simulink model "SingleTrack"  (R2019b)
settings: Solver=ode1  StartTime=0  StopTime=250  FixedStep=1.0000000000000000e-003  RelTol=1e-3
InitFcn:
  | sampleTime = str2double(get_param(bdroot, 'FixedStep'));
undefined symbols (not defined in the file or in its folder): AccPedalPos, BrakePedalPos, BrakeSwitch, DiscIntNeverNeededParam, DYNA4, EngSpd, IgnitionSwitch, InitialGear, InitialSpeed, IntendedEngTrq, LeftIndicator, MainBrakePress, MaxGear, MDL, MinGear, RefAcc, RefLane, RefLatPos, RefPath, RefPathCurv, RefSpd, RefSpdPreview, RefSpdRetrospect, RightIndicator, SteeringWheelAng, SteeringWheelTrq, UserDefinedRefValue, vm_const
libraries: UtilitiesLibrary x31, simulink x18, WheelSystemModules x13, LongitudinalControllerModules x13, LateralControllerModules x7, AnimationBusselectorModules x5, EnvironmentModules x5, BasicEngineControlModules x5, MiscellaneousControlModules x5, Animation3Modules x4, AuxiliariesModules x4, ReducedTireModules x4
(part 31 of 32)

== system SingleTrack/VehicleControl/LongitudinalControl/ControlSystemsPreprocessor/Generation of Hold Data/Enabled Subsystem ==
  LongCTRL : Inport
  VehicleInfo : Inport  Port=2
  Enable : EnablePort  StatesWhenEnabling=reset  PropagateVarSize=During execution
  Add : Sum  Inputs=+-
  All zeros TD_BO_LongitudinalControlInputs : Constant  Value=0  OutDataTypeStr=Bus: TD_BO_LongitudinalControlInputs
  Bus Assignment : BusAssignment  AssignedSignals=AccPedalPos,BrakePedalPos,MainBrakePress,FrontLeftWheelBrakePress,FrontRightWheelBrakePress,RearLeftWheelBrakePress,RearRightWheelBrakePress,Rear2LeftWheelBrakePress,Rear2RightWheelBrakePress,Rear3LeftWheelBrakePress,Rear3RightWheelBrakePress,TrailerFrontLeftWheelBrakePress,TrailerFrontRightWheelBrakePress,TrailerRearLeftWheelBrakePress,TrailerRearRightWheelBrakePress,TrailerRear2LeftWheelBrakePress,TrailerRear2RightWheelBrakePress,TrailerRear3LeftWheelBrakePress,TrailerRear3RightWheelBrakePress,MinGear,MaxGear,ClutchPedalPos,ShiftingProgramSelection,IgnitionSwitch,Handbrake,ParkingLock,FrontDifferentialLock,RearDifferentialLock,Rear2DifferentialLock,Rear3DifferentialLock,TransferCaseLock,DayRunningLight,LowBeamLight,HighBeamLight,FogLampFront,FogLampRear,ESCSwitch,ABSSwitch,ACCSwitch,ACCRefSpd,AEBSwitch,RefSpd,RefSpdPreview,RefSpdRetrospect,RefAcc
  Bus Selector1 : BusSelector  OutputSignals=Chassis_VehicleBody_AbsVel[m/s],Chassis_VehicleBody_Acc_wrt_WorldSys(VehSys)[m/s**2]
  Bus Selector15 : BusSelector  OutputSignals=AccPedalPos[0_1],BrakePedalPos[0_1],MainBrakePress[Pa],FrontLeftWheelBrakePress[Pa],FrontRightWheelBrakePress[Pa],RearLeftWheelBrakePress[Pa],RearRightWheelBrakePress[Pa],Rear2LeftWheelBrakePress[Pa],Rear2RightWheelBrakePress[Pa],Rear3LeftWheelBrakePress[Pa],Rear3RightWheelBrakePress[Pa],TrailerFrontLeftWheelBrakePress[Pa],TrailerFrontRightWheelBrakePress[Pa],TrailerRearLeftWheelBrakePress[Pa],TrailerRearRightWheelBrakePress[Pa],TrailerRear2LeftWheelBrakePress[Pa],TrailerRear2RightWheelBrakePress[Pa],TrailerRear3LeftWheelBrakePress[Pa],TrailerRear3RightWheelBrakePress[Pa],MinGear[-4;20],MaxGear[-4;20],ClutchPos[0_1],ShiftingProgramSelection[-],IgnitionSwitch[0;3],Handbrake[0_1],ParkingLock[0;1],FrontDifferentialLock[0;1],RearDifferentialLock[0;1],Rear2DifferentialLock[0;1],Rear3DifferentialLock[0;1],TransferCaseLock[0;1],DayRunningLight[0;1],LowBeamLight[0;1],HighBeamLight[0;1],FogLampFront[0;1],FogLampRear[0;1],ESCSwitch[0;1],ABSSwitch[0;1],ACCSwitch[0;1],ACCRefSpd[m/s],AEBSwitch[0;1]
  Constant1 : Constant
  y component : Selector  InputPortWidth=3  IndexOptions=Index vector (dialog)  Indices=1  OutputSizes=1
  HoldData : Outport  VectorParamsAs1DForOutWhenUnconnected=off
  wires:
  Bus Selector15/21 -> Bus Assignment/22  "<MaxGear[-4;20]>"
  Bus Selector15/20 -> Bus Assignment/21  "<MinGear[-4;20]>"
  Bus Selector15/22 -> Add/2  "<ClutchPos[0_1]>"
  Bus Selector15/29 -> Bus Assignment/30  "<Rear2DifferentialLock[0;1]>"
  Bus Selector15/31 -> Bus Assignment/32  "<TransferCaseLock[0;1]>"
  Bus Selector15/6 -> Bus Assignment/7  "<RearLeftWheelBrakePress[Pa]>"
  Bus Selector15/28 -> Bus Assignment/29  "<RearDifferentialLock[0;1]>"
  Bus Selector15/17 -> Bus Assignment/18  "<TrailerRear2RightWheelBrakePress[Pa]>"
  Bus Selector15/36 -> Bus Assignment/37  "<FogLampRear[0;1]>"
  Bus Selector15/30 -> Bus Assignment/31  "<Rear3DifferentialLock[0;1]>"
  Bus Selector15/13 -> Bus Assignment/14  "<TrailerFrontRightWheelBrakePress[Pa]>"
  Bus Selector15/35 -> Bus Assignment/36  "<FogLampFront[0;1]>"
  Bus Selector15/2 -> Bus Assignment/3  "<BrakePedalPos[0_1]>"
  Bus Selector15/16 -> Bus Assignment/17  "<TrailerRear2LeftWheelBrakePress[Pa]>"
  Bus Selector15/15 -> Bus Assignment/16  "<TrailerRearRightWheelBrakePress[Pa]>"
  Bus Selector15/9 -> Bus Assignment/10  "<Rear2RightWheelBrakePress[Pa]>"
  Bus Selector15/19 -> Bus Assignment/20  "<TrailerRear3RightWheelBrakePress[Pa]>"
  Bus Selector15/23 -> Bus Assignment/24  "<ShiftingProgramSelection[-]>"
  Bus Selector15/8 -> Bus Assignment/9  "<Rear2LeftWheelBrakePress[Pa]>"
  Bus Selector15/34 -> Bus Assignment/35  "<HighBeamLight[0;1]>"
  Bus Selector15/24 -> Bus Assignment/25  "<IgnitionSwitch[0;3]>"
  Bus Selector15/33 -> Bus Assignment/34  "<LowBeamLight[0;1]>"
  Bus Selector15/26 -> Bus Assignment/27  "<ParkingLock[0;1]>"
  Bus Selector15/25 -> Bus Assignment/26  "<Handbrake[0_1]>"
  Bus Selector15/12 -> Bus Assignment/13  "<TrailerFrontLeftWheelBrakePress[Pa]>"
  Bus Selector15/10 -> Bus Assignment/11  "<Rear3LeftWheelBrakePress[Pa]>"
  Bus Selector15/14 -> Bus Assignment/15  "<TrailerRearLeftWheelBrakePress[Pa]>"
  Bus Selector15/7 -> Bus Assignment/8  "<RearRightWheelBrakePress[Pa]>"
  Bus Selector15/5 -> Bus Assignment/6  "<FrontRightWheelBrakePress[Pa]>"
  Bus Selector15/1 -> Bus Assignment/2  "<AccPedalPos[0_1]>"
  Bus Selector15/32 -> Bus Assignment/33  "<DayRunningLight[0;1]>"
  Bus Selector15/11 -> Bus Assignment/12  "<Rear3RightWheelBrakePress[Pa]>"
  Bus Selector15/3 -> Bus Assignment/4  "<MainBrakePress[Pa]>"
  Bus Selector15/27 -> Bus Assignment/28  "<FrontDifferentialLock[0;1]>"
  Bus Selector15/4 -> Bus Assignment/5  "<FrontLeftWheelBrakePress[Pa]>"
  Bus Selector15/18 -> Bus Assignment/19  "<TrailerRear3LeftWheelBrakePress[Pa]>"
  Bus Selector15/39 -> Bus Assignment/40  "<ACCSwitch[0;1]>"
  Bus Selector15/37 -> Bus Assignment/38  "<ESCSwitch[0;1]>"
  Bus Selector15/38 -> Bus Assignment/39  "<ABSSwitch[0;1]>"
  All zeros TD_BO_LongitudinalControlInputs/1 -> Bus Assignment/1
  Bus Selector15/40 -> Bus Assignment/41  "<ACCRefSpd[m/s]>"
  Bus Selector15/41 -> Bus Assignment/42  "<AEBSwitch[0;1]>"
  Bus Selector1/2 -> y component/1  "<Chassis_VehicleBody_Acc_wrt_WorldSys(VehSys)[m/s**2]>"
  Constant1/1 -> Add/1
  y component/1 -> Bus Assignment/46  "RefAcc"
  LongCTRL/1 -> Bus Selector15/1
  VehicleInfo/1 -> Bus Selector1/1
  Bus Assignment/1 -> HoldData/1
  Add/1 -> Bus Assignment/23  "ClutchPedalPos[0_1]"
  Bus Selector1/1 -> Bus Assignment/45, Bus Assignment/44, Bus Assignment/43  "<Chassis_VehicleBody_AbsVel[m/s]>"

== system SingleTrack/VehicleControl/LongitudinalControl/ControlSystemsPreprocessor/Generation of Hold Data/InitialAction Subsystem ==
  LongitudinalControlInputs : Inport
  Action Port : ActionPort  InitializeStates=reset  ActionPortLabel=case [ 1 ]:
  All zeros TD_BO_LongitudinalControlInputs : Constant  Value=0  OutDataTypeStr=Bus: TD_BO_LongitudinalControlInputs
  Bus Assignment : BusAssignment  AssignedSignals=InitialSpeed,RefSpd,RefSpdPreview,RefSpdRetrospect,InitialGear,MinGear,MaxGear
  Bus Selector1 : BusSelector  OutputSignals=InitialSpeed,InitialGear
  InitialLongitudinalControlInputs : Outport  VectorParamsAs1DForOutWhenUnconnected=off
  wires:
  Bus Selector1/2 -> Bus Assignment/6, Bus Assignment/7, Bus Assignment/8  "<InitialGear>"
  All zeros TD_BO_LongitudinalControlInputs/1 -> Bus Assignment/1
  Bus Selector1/1 -> Bus Assignment/5, Bus Assignment/4, Bus Assignment/3, Bus Assignment/2  "<InitialSpeed>"
  Bus Assignment/1 -> InitialLongitudinalControlInputs/1
  LongitudinalControlInputs/1 -> Bus Selector1/1

== system SingleTrack/VehicleControl/LongitudinalControl/ControlSystemsPreprocessor/Generation of Speed Data/Smooth Derivative ==
  note: This transfer function calculates a smooth acceleration with continuous jerk from a speed input signal.
      | The smoothing time constant T = previewTime / 2 is an input signal.
  RefSpdPrev[m/s] : Inport
  PreviewTime[s] : Inport  Port=2
  Enable : EnablePort  StatesWhenEnabling=reset
  Gain1 : Gain  Gain=0.5
  Max : MinMax  Function=max  Inputs=2
  Transfer Fcn with variable prameter : Subsystem
      mask Display: disp('num = s \n den = T^2*s^2 + 2*T*s + 1')
  limit to +/-20 : Saturate  UpperLimit=20  LowerLimit=-20
  minimum smoothing constant : Constant  Value=0.01
  SmoothedRefAcc[m/s**2] : Outport  OutputWhenDisabled=reset  InitialOutput=0  VectorParamsAs1DForOutWhenUnconnected=off
  wires:
  PreviewTime[s]/1 -> Gain1/1
  minimum smoothing constant/1 -> Max/2
  Gain1/1 -> Max/1
  RefSpdPrev[m/s]/1 -> Transfer Fcn with variable prameter/1(u)
  Max/1 -> Transfer Fcn with variable prameter/2(T)
  Transfer Fcn with variable prameter/1(y) -> limit to +/-20/1
  limit to +/-20/1 -> SmoothedRefAcc[m/s**2]/1

== system SingleTrack/VehicleControl/LongitudinalControl/ControlSystemsPreprocessor/Generation of Speed Data/Target Speed Computation Check ==
  note: TASK_LONG_ACC_BRAKE_INPUTS = 1;
      | TASK_LONG_SPEED_CONTROL = 2;
      | TASK_LONG_ACCELERATION_CONTROL = 3;
      | TASK_LONG_USER_DEFINED = 4;
  note: SOURCE_NOMINALPATH = 1;
      | 	SOURCE_LANE = 2;
      | 	SOURCE_CONSTANT = 3;
      | 	SOURCE_TABLE_DISCRETE = 4;
      | 	SOURCE_TABLE_LINEAR = 5;
      | 	SOURCE_TABLE_CUBIC = 6;
      | 	SOURCE_TABLE_HAVERSINE = 7;
      | 	SOURCE_AUTOMATIC = 8;
      | 	SOURCE_SINE_TIME = 9;
      | 	SOURCE_SINE_PATH = 10;
      | 	SOURCE_HOLD = 11;
      | 	SOURCE_EXTERNAL = 12;
      | 	SOURCE_EXTERNAL_NOMINALPATH = 13;
      | 	SOURCE_EXTERNAL_LANE = 14;
  TaskIdentifiers : Inport
  SourceIdentifiers : Inport  Port=2
  Bus Selector : BusSelector  OutputSignals=RefSpd
  Bus Selector1 : BusSelector  OutputSignals=Task
  Compare To Constant : simulink/Logic and Bit Operations/Compare To Constant  relop===  const=vm_const('TASK_LONG_SPEED_CONTROL')  OutDataTypeStr=boolean  ZeroCross=off
  Compare To Constant1 : simulink/Logic and Bit Operations/Compare To Constant  relop===  const=vm_const('SOURCE_AUTOMATIC')  OutDataTypeStr=uint8  ZeroCross=off
  Compare To Constant2 : simulink/Logic and Bit Operations/Compare To Constant  relop===  const=vm_const('TASK_LONG_USER_DEFINED')  OutDataTypeStr=boolean  ZeroCross=off
  Compare To Constant3 : simulink/Logic and Bit Operations/Compare To Constant  relop===  const=vm_const('TASK_LONG_ACCELERATION_CONTROL')  OutDataTypeStr=boolean  ZeroCross=off
  Data Type Conversion : DataTypeConversion  OutDataTypeStr=int8
  Logical Operator : Logic  AllPortsSameDT=off
  Logical Operator1 : Logic  Operator=OR  AllPortsSameDT=off
  Logical Operator3 : Logic  AllPortsSameDT=off
  Logical Operator4 : Logic  Operator=NOT  AllPortsSameDT=off
  isAutomatic : Outport  VectorParamsAs1DForOutWhenUnconnected=off
  isAccelerationControl : Outport  Port=2  VectorParamsAs1DForOutWhenUnconnected=off
  needsSmoothedDerivative : Outport  Port=3  VectorParamsAs1DForOutWhenUnconnected=off
  wires:
  Compare To Constant3/1 -> isAccelerationControl/1
  Data Type Conversion/1 -> Compare To Constant1/1
  Logical Operator1/1 -> Logical Operator/1
  Compare To Constant/1 -> Logical Operator3/1, Logical Operator1/1
  Compare To Constant2/1 -> Logical Operator1/2
  Logical Operator/1 -> isAutomatic/1
  Compare To Constant1/1 -> Logical Operator4/1, Logical Operator/2
  SourceIdentifiers/1 -> Bus Selector/1
  Bus Selector/1 -> Data Type Conversion/1  "<RefSpd>"
  Bus Selector1/1 -> Compare To Constant2/1, Compare To Constant/1, Compare To Constant3/1  "<Task>"
  TaskIdentifiers/1 -> Bus Selector1/1
  Logical Operator4/1 -> Logical Operator3/2
  Logical Operator3/1 -> needsSmoothedDerivative/1

== system SingleTrack/Vehicle/Drivetrain/DrivetrainPhysics/DrivetrainPhysicsOutputs/ClutchOutput/ClutchOutput ==
  Trq[Nm]___UNIQUE_1 : Inport  Description=|  PortDimensions=[1]
      | <name>Trq[Nm]</name>
      | <comment></comment>
  Pos[0_1]___UNIQUE_1 : Inport  Description=|  Port=2  PortDimensions=[1]
      | <name>Pos[0_1]</name>
      | <comment></comment>
  __TDD__Clutch.Pos[0_1] : Demux  Outputs=[1]
  __TDD__Clutch.Trq[Nm] : Demux  Outputs=[1]
  __TDO__Clutch : BusCreator  Inputs=2
  Clutch___UNIQUE_1 : Outport  Description=|  PortDimensions=[2]  VectorParamsAs1DForOutWhenUnconnected=off
      | <name>Trq[Nm]</name>
      | <comment></comment>
  wires:
  __TDO__Clutch/1 -> Clutch___UNIQUE_1/1  "Clutch"
  __TDD__Clutch.Pos[0_1]/1 -> __TDO__Clutch/2  "Pos[0_1]"
  Pos[0_1]___UNIQUE_1/1 -> __TDD__Clutch.Pos[0_1]/1
  __TDD__Clutch.Trq[Nm]/1 -> __TDO__Clutch/1  "Trq[Nm]"
  Trq[Nm]___UNIQUE_1/1 -> __TDD__Clutch.Trq[Nm]/1

== system SingleTrack/Vehicle/Drivetrain/DrivetrainPhysics/DrivetrainPhysicsOutputs/FrontDifferentialOutput/FrontDifferentialOutput ==
  TrqDistributionFac[0_1]___UNIQUE_1 : Inport  Description=|  PortDimensions=[1]
      | <name>TrqDistributionFac[0_1]</name>
      | <comment></comment>
  __TDD__FrontDifferential.TrqDistributionFac[0_1] : Demux  Outputs=[1]
  __TDO__FrontDifferential : BusCreator  Inputs=1
  FrontDifferential___UNIQUE_1 : Outport  Description=|  PortDimensions=[1]  VectorParamsAs1DForOutWhenUnconnected=off
      | <name>TrqDistributionFac[0_1]</name>
      | <comment></comment>
  wires:
  __TDO__FrontDifferential/1 -> FrontDifferential___UNIQUE_1/1  "FrontDifferential"
  __TDD__FrontDifferential.TrqDistributionFac[0_1]/1 -> __TDO__FrontDifferential/1  "TrqDistributionFac[0_1]"
  TrqDistributionFac[0_1]___UNIQUE_1/1 -> __TDD__FrontDifferential.TrqDistributionFac[0_1]/1

== system SingleTrack/Vehicle/Drivetrain/DrivetrainPhysics/DrivetrainPhysicsOutputs/FrontLeftShaftOutput/FrontLeftShaftOutput ==
  Trq[Nm]___UNIQUE_1 : Inport  Description=|  PortDimensions=[1]
      | <name>Trq[Nm]</name>
      | <comment></comment>
  RotSpdDifferentialOut[rad/s]___UNIQUE_1 : Inport  Description=|  Port=2  PortDimensions=[1]
      | <name>RotSpdDifferentialOut[rad/s]</name>
      | <comment></comment>
  RotAcc[rad/s**2]___UNIQUE_1 : Inport  Description=|  Port=3  PortDimensions=[1]
      | <name>RotAcc[rad/s**2]</name>
      | <comment></comment>
  DerivativeOfTrq_wrt_RotAng[Nm/rad]___UNIQUE_1 : Inport  Description=|  Port=4  PortDimensions=[1]
      | <name>DerivativeOfTrq_wrt_RotAng[Nm/rad]</name>
      | <comment></comment>
  DerivativeOfTrq_wrt_WheelSpd[Nm/(rad/s)]___UNIQUE_1 : Inport  Description=|  Port=5  PortDimensions=[1]
      | <name>DerivativeOfTrq_wrt_WheelSpd[Nm/(rad/s)]</name>
      | <comment></comment>
  AddInrt[kg*m**2]___UNIQUE_1 : Inport  Description=|  Port=6  PortDimensions=[1]
      | <name>AddInrt[kg*m**2]</name>
      | <comment></comment>
  FrictionTrq[Nm]___UNIQUE_1 : Inport  Description=|  Port=7  PortDimensions=[1]
      | <name>FrictionTrq[Nm]</name>
      | <comment></comment>
  __TDD__FrontLeftShaft.AddInrt[kg*m**2] : Demux  Outputs=[1]
  __TDD__FrontLeftShaft.DerivativeOfTrq_wrt_RotAng[Nm/rad] : Demux  Outputs=[1]
  __TDD__FrontLeftShaft.DerivativeOfTrq_wrt_WheelSpd[Nm/(rad/s)] : Demux  Outputs=[1]
  __TDD__FrontLeftShaft.FrictionTrq[Nm] : Demux  Outputs=[1]
  __TDD__FrontLeftShaft.RotAcc[rad/s**2] : Demux  Outputs=[1]
  __TDD__FrontLeftShaft.RotSpdDifferentialOut[rad/s] : Demux  Outputs=[1]
  __TDD__FrontLeftShaft.Trq[Nm] : Demux  Outputs=[1]
  __TDO__FrontLeftShaft : BusCreator  Inputs=7
  FrontLeftShaft___UNIQUE_1 : Outport  Description=|  PortDimensions=[7]  VectorParamsAs1DForOutWhenUnconnected=off
      | <name>Trq[Nm]</name>
      | <comment></comment>
  wires:
  __TDO__FrontLeftShaft/1 -> FrontLeftShaft___UNIQUE_1/1  "FrontLeftShaft"
  __TDD__FrontLeftShaft.FrictionTrq[Nm]/1 -> __TDO__FrontLeftShaft/7  "FrictionTrq[Nm]"
  FrictionTrq[Nm]___UNIQUE_1/1 -> __TDD__FrontLeftShaft.FrictionTrq[Nm]/1
  __TDD__FrontLeftShaft.AddInrt[kg*m**2]/1 -> __TDO__FrontLeftShaft/6  "AddInrt[kg*m**2]"
  AddInrt[kg*m**2]___UNIQUE_1/1 -> __TDD__FrontLeftShaft.AddInrt[kg*m**2]/1
  __TDD__FrontLeftShaft.DerivativeOfTrq_wrt_WheelSpd[Nm/(rad/s)]/1 -> __TDO__FrontLeftShaft/5  "DerivativeOfTrq_wrt_WheelSpd[Nm/(rad/s)]"
  DerivativeOfTrq_wrt_WheelSpd[Nm/(rad/s)]___UNIQUE_1/1 -> __TDD__FrontLeftShaft.DerivativeOfTrq_wrt_WheelSpd[Nm/(rad/s)]/1
  __TDD__FrontLeftShaft.DerivativeOfTrq_wrt_RotAng[Nm/rad]/1 -> __TDO__FrontLeftShaft/4  "DerivativeOfTrq_wrt_RotAng[Nm/rad]"
  DerivativeOfTrq_wrt_RotAng[Nm/rad]___UNIQUE_1/1 -> __TDD__FrontLeftShaft.DerivativeOfTrq_wrt_RotAng[Nm/rad]/1
  __TDD__FrontLeftShaft.RotAcc[rad/s**2]/1 -> __TDO__FrontLeftShaft/3  "RotAcc[rad/s**2]"
  RotAcc[rad/s**2]___UNIQUE_1/1 -> __TDD__FrontLeftShaft.RotAcc[rad/s**2]/1
  __TDD__FrontLeftShaft.RotSpdDifferentialOut[rad/s]/1 -> __TDO__FrontLeftShaft/2  "RotSpdDifferentialOut[rad/s]"
  RotSpdDifferentialOut[rad/s]___UNIQUE_1/1 -> __TDD__FrontLeftShaft.RotSpdDifferentialOut[rad/s]/1
  __TDD__FrontLeftShaft.Trq[Nm]/1 -> __TDO__FrontLeftShaft/1  "Trq[Nm]"
  Trq[Nm]___UNIQUE_1/1 -> __TDD__FrontLeftShaft.Trq[Nm]/1

== system SingleTrack/Vehicle/Drivetrain/DrivetrainPhysics/DrivetrainPhysicsOutputs/FrontRightShaftOutput/FrontRightShaftOutput ==
  Trq[Nm]___UNIQUE_1 : Inport  Description=|  PortDimensions=[1]
      | <name>Trq[Nm]</name>
      | <comment></comment>
  RotSpdDifferentialOut[rad/s]___UNIQUE_1 : Inport  Description=|  Port=2  PortDimensions=[1]
      | <name>RotSpdDifferentialOut[rad/s]</name>
      | <comment></comment>
  RotAcc[rad/s**2]___UNIQUE_1 : Inport  Description=|  Port=3  PortDimensions=[1]
      | <name>RotAcc[rad/s**2]</name>
      | <comment></comment>
  DerivativeOfTrq_wrt_RotAng[Nm/rad]___UNIQUE_1 : Inport  Description=|  Port=4  PortDimensions=[1]
      | <name>DerivativeOfTrq_wrt_RotAng[Nm/rad]</name>
      | <comment></comment>
  DerivativeOfTrq_wrt_WheelSpd[Nm/(rad/s)]___UNIQUE_1 : Inport  Description=|  Port=5  PortDimensions=[1]
      | <name>DerivativeOfTrq_wrt_WheelSpd[Nm/(rad/s)]</name>
      | <comment></comment>
  AddInrt[kg*m**2]___UNIQUE_1 : Inport  Description=|  Port=6  PortDimensions=[1]
      | <name>AddInrt[kg*m**2]</name>
      | <comment></comment>
  FrictionTrq[Nm]___UNIQUE_1 : Inport  Description=|  Port=7  PortDimensions=[1]
      | <name>FrictionTrq[Nm]</name>
      | <comment></comment>
  __TDD__FrontRightShaft.AddInrt[kg*m**2] : Demux  Outputs=[1]
  __TDD__FrontRightShaft.DerivativeOfTrq_wrt_RotAng[Nm/rad] : Demux  Outputs=[1]
  __TDD__FrontRightShaft.DerivativeOfTrq_wrt_WheelSpd[Nm/(rad/s)] : Demux  Outputs=[1]
  __TDD__FrontRightShaft.FrictionTrq[Nm] : Demux  Outputs=[1]
  __TDD__FrontRightShaft.RotAcc[rad/s**2] : Demux  Outputs=[1]
  __TDD__FrontRightShaft.RotSpdDifferentialOut[rad/s] : Demux  Outputs=[1]
  __TDD__FrontRightShaft.Trq[Nm] : Demux  Outputs=[1]
  __TDO__FrontRightShaft : BusCreator  Inputs=7
  FrontRightShaft___UNIQUE_1 : Outport  Description=|  PortDimensions=[7]  VectorParamsAs1DForOutWhenUnconnected=off
      | <name>Trq[Nm]</name>
      | <comment></comment>
  wires:
  __TDO__FrontRightShaft/1 -> FrontRightShaft___UNIQUE_1/1  "FrontRightShaft"
  __TDD__FrontRightShaft.FrictionTrq[Nm]/1 -> __TDO__FrontRightShaft/7  "FrictionTrq[Nm]"
  FrictionTrq[Nm]___UNIQUE_1/1 -> __TDD__FrontRightShaft.FrictionTrq[Nm]/1
  __TDD__FrontRightShaft.AddInrt[kg*m**2]/1 -> __TDO__FrontRightShaft/6  "AddInrt[kg*m**2]"
  AddInrt[kg*m**2]___UNIQUE_1/1 -> __TDD__FrontRightShaft.AddInrt[kg*m**2]/1
  __TDD__FrontRightShaft.DerivativeOfTrq_wrt_WheelSpd[Nm/(rad/s)]/1 -> __TDO__FrontRightShaft/5  "DerivativeOfTrq_wrt_WheelSpd[Nm/(rad/s)]"
  DerivativeOfTrq_wrt_WheelSpd[Nm/(rad/s)]___UNIQUE_1/1 -> __TDD__FrontRightShaft.DerivativeOfTrq_wrt_WheelSpd[Nm/(rad/s)]/1
  __TDD__FrontRightShaft.DerivativeOfTrq_wrt_RotAng[Nm/rad]/1 -> __TDO__FrontRightShaft/4  "DerivativeOfTrq_wrt_RotAng[Nm/rad]"
  DerivativeOfTrq_wrt_RotAng[Nm/rad]___UNIQUE_1/1 -> __TDD__FrontRightShaft.DerivativeOfTrq_wrt_RotAng[Nm/rad]/1
  __TDD__FrontRightShaft.RotAcc[rad/s**2]/1 -> __TDO__FrontRightShaft/3  "RotAcc[rad/s**2]"
  RotAcc[rad/s**2]___UNIQUE_1/1 -> __TDD__FrontRightShaft.RotAcc[rad/s**2]/1
  __TDD__FrontRightShaft.RotSpdDifferentialOut[rad/s]/1 -> __TDO__FrontRightShaft/2  "RotSpdDifferentialOut[rad/s]"
  RotSpdDifferentialOut[rad/s]___UNIQUE_1/1 -> __TDD__FrontRightShaft.RotSpdDifferentialOut[rad/s]/1
  __TDD__FrontRightShaft.Trq[Nm]/1 -> __TDO__FrontRightShaft/1  "Trq[Nm]"
  Trq[Nm]___UNIQUE_1/1 -> __TDD__FrontRightShaft.Trq[Nm]/1

== system SingleTrack/Vehicle/Drivetrain/DrivetrainPhysics/DrivetrainPhysicsOutputs/RearDifferentialOutput/RearDifferentialOutput ==
  TrqDistributionFac[0_1]___UNIQUE_1 : Inport  Description=|  PortDimensions=[1]
      | <name>TrqDistributionFac[0_1]</name>
      | <comment></comment>
  __TDD__RearDifferential.TrqDistributionFac[0_1] : Demux  Outputs=[1]
  __TDO__RearDifferential : BusCreator  Inputs=1
  RearDifferential___UNIQUE_1 : Outport  Description=|  PortDimensions=[1]  VectorParamsAs1DForOutWhenUnconnected=off
      | <name>TrqDistributionFac[0_1]</name>
      | <comment></comment>
  wires:
  __TDO__RearDifferential/1 -> RearDifferential___UNIQUE_1/1  "RearDifferential"
  __TDD__RearDifferential.TrqDistributionFac[0_1]/1 -> __TDO__RearDifferential/1  "TrqDistributionFac[0_1]"
  TrqDistributionFac[0_1]___UNIQUE_1/1 -> __TDD__RearDifferential.TrqDistributionFac[0_1]/1

== system SingleTrack/Vehicle/Drivetrain/DrivetrainPhysics/DrivetrainPhysicsOutputs/RearLeftShaftOutput/RearLeftShaftOutput ==
  Trq[Nm]___UNIQUE_1 : Inport  Description=|  PortDimensions=[1]
      | <name>Trq[Nm]</name>
      | <comment></comment>
  RotSpdDifferentialOut[rad/s]___UNIQUE_1 : Inport  Description=|  Port=2  PortDimensions=[1]
      | <name>RotSpdDifferentialOut[rad/s]</name>
      | <comment></comment>
  RotAcc[rad/s**2]___UNIQUE_1 : Inport  Description=|  Port=3  PortDimensions=[1]
      | <name>RotAcc[rad/s**2]</name>
      | <comment></comment>
  DerivativeOfTrq_wrt_RotAng[Nm/rad]___UNIQUE_1 : Inport  Description=|  Port=4  PortDimensions=[1]
      | <name>DerivativeOfTrq_wrt_RotAng[Nm/rad]</name>
      | <comment></comment>
  DerivativeOfTrq_wrt_WheelSpd[Nm/(rad/s)]___UNIQUE_1 : Inport  Description=|  Port=5  PortDimensions=[1]
      | <name>DerivativeOfTrq_wrt_WheelSpd[Nm/(rad/s)]</name>
      | <comment></comment>
  AddInrt[kg*m**2]___UNIQUE_1 : Inport  Description=|  Port=6  PortDimensions=[1]
      | <name>AddInrt[kg*m**2]</name>
      | <comment></comment>
  FrictionTrq[Nm]___UNIQUE_1 : Inport  Description=|  Port=7  PortDimensions=[1]
      | <name>FrictionTrq[Nm]</name>
      | <comment></comment>
  __TDD__RearLeftShaft.AddInrt[kg*m**2] : Demux  Outputs=[1]
  __TDD__RearLeftShaft.DerivativeOfTrq_wrt_RotAng[Nm/rad] : Demux  Outputs=[1]
  __TDD__RearLeftShaft.DerivativeOfTrq_wrt_WheelSpd[Nm/(rad/s)] : Demux  Outputs=[1]
  __TDD__RearLeftShaft.FrictionTrq[Nm] : Demux  Outputs=[1]
  __TDD__RearLeftShaft.RotAcc[rad/s**2] : Demux  Outputs=[1]
  __TDD__RearLeftShaft.RotSpdDifferentialOut[rad/s] : Demux  Outputs=[1]
  __TDD__RearLeftShaft.Trq[Nm] : Demux  Outputs=[1]
  __TDO__RearLeftShaft : BusCreator  Inputs=7
  RearLeftShaft___UNIQUE_1 : Outport  Description=|  PortDimensions=[7]  VectorParamsAs1DForOutWhenUnconnected=off
      | <name>Trq[Nm]</name>
      | <comment></comment>
  wires:
  __TDO__RearLeftShaft/1 -> RearLeftShaft___UNIQUE_1/1  "RearLeftShaft"
  __TDD__RearLeftShaft.FrictionTrq[Nm]/1 -> __TDO__RearLeftShaft/7  "FrictionTrq[Nm]"
  FrictionTrq[Nm]___UNIQUE_1/1 -> __TDD__RearLeftShaft.FrictionTrq[Nm]/1
  __TDD__RearLeftShaft.AddInrt[kg*m**2]/1 -> __TDO__RearLeftShaft/6  "AddInrt[kg*m**2]"
  AddInrt[kg*m**2]___UNIQUE_1/1 -> __TDD__RearLeftShaft.AddInrt[kg*m**2]/1
  __TDD__RearLeftShaft.DerivativeOfTrq_wrt_WheelSpd[Nm/(rad/s)]/1 -> __TDO__RearLeftShaft/5  "DerivativeOfTrq_wrt_WheelSpd[Nm/(rad/s)]"
  DerivativeOfTrq_wrt_WheelSpd[Nm/(rad/s)]___UNIQUE_1/1 -> __TDD__RearLeftShaft.DerivativeOfTrq_wrt_WheelSpd[Nm/(rad/s)]/1
  __TDD__RearLeftShaft.DerivativeOfTrq_wrt_RotAng[Nm/rad]/1 -> __TDO__RearLeftShaft/4  "DerivativeOfTrq_wrt_RotAng[Nm/rad]"
  DerivativeOfTrq_wrt_RotAng[Nm/rad]___UNIQUE_1/1 -> __TDD__RearLeftShaft.DerivativeOfTrq_wrt_RotAng[Nm/rad]/1
  __TDD__RearLeftShaft.RotAcc[rad/s**2]/1 -> __TDO__RearLeftShaft/3  "RotAcc[rad/s**2]"
  RotAcc[rad/s**2]___UNIQUE_1/1 -> __TDD__RearLeftShaft.RotAcc[rad/s**2]/1
  __TDD__RearLeftShaft.RotSpdDifferentialOut[rad/s]/1 -> __TDO__RearLeftShaft/2  "RotSpdDifferentialOut[rad/s]"
  RotSpdDifferentialOut[rad/s]___UNIQUE_1/1 -> __TDD__RearLeftShaft.RotSpdDifferentialOut[rad/s]/1
  __TDD__RearLeftShaft.Trq[Nm]/1 -> __TDO__RearLeftShaft/1  "Trq[Nm]"
  Trq[Nm]___UNIQUE_1/1 -> __TDD__RearLeftShaft.Trq[Nm]/1

== system SingleTrack/Vehicle/Drivetrain/DrivetrainPhysics/DrivetrainPhysicsOutputs/RearRightShaftOutput/RearRightShaftOutput ==
  Trq[Nm]___UNIQUE_1 : Inport  Description=|  PortDimensions=[1]
      | <name>Trq[Nm]</name>
      | <comment></comment>
  RotSpdDifferentialOut[rad/s]___UNIQUE_1 : Inport  Description=|  Port=2  PortDimensions=[1]
      | <name>RotSpdDifferentialOut[rad/s]</name>
      | <comment></comment>
  RotAcc[rad/s**2]___UNIQUE_1 : Inport  Description=|  Port=3  PortDimensions=[1]
      | <name>RotAcc[rad/s**2]</name>
      | <comment></comment>
  DerivativeOfTrq_wrt_RotAng[Nm/rad]___UNIQUE_1 : Inport  Description=|  Port=4  PortDimensions=[1]
      | <name>DerivativeOfTrq_wrt_RotAng[Nm/rad]</name>
      | <comment></comment>
  DerivativeOfTrq_wrt_WheelSpd[Nm/(rad/s)]___UNIQUE_1 : Inport  Description=|  Port=5  PortDimensions=[1]
      | <name>DerivativeOfTrq_wrt_WheelSpd[Nm/(rad/s)]</name>
      | <comment></comment>
  AddInrt[kg*m**2]___UNIQUE_1 : Inport  Description=|  Port=6  PortDimensions=[1]
      | <name>AddInrt[kg*m**2]</name>
      | <comment></comment>
  FrictionTrq[Nm]___UNIQUE_1 : Inport  Description=|  Port=7  PortDimensions=[1]
      | <name>FrictionTrq[Nm]</name>
      | <comment></comment>
  __TDD__RearRightShaft.AddInrt[kg*m**2] : Demux  Outputs=[1]
  __TDD__RearRightShaft.DerivativeOfTrq_wrt_RotAng[Nm/rad] : Demux  Outputs=[1]
  __TDD__RearRightShaft.DerivativeOfTrq_wrt_WheelSpd[Nm/(rad/s)] : Demux  Outputs=[1]
  __TDD__RearRightShaft.FrictionTrq[Nm] : Demux  Outputs=[1]
  __TDD__RearRightShaft.RotAcc[rad/s**2] : Demux  Outputs=[1]
  __TDD__RearRightShaft.RotSpdDifferentialOut[rad/s] : Demux  Outputs=[1]
  __TDD__RearRightShaft.Trq[Nm] : Demux  Outputs=[1]
  __TDO__RearRightShaft : BusCreator  Inputs=7
  RearRightShaft___UNIQUE_1 : Outport  Description=|  PortDimensions=[7]  VectorParamsAs1DForOutWhenUnconnected=off
      | <name>Trq[Nm]</name>
      | <comment></comment>
  wires:
  __TDO__RearRightShaft/1 -> RearRightShaft___UNIQUE_1/1  "RearRightShaft"
  __TDD__RearRightShaft.FrictionTrq[Nm]/1 -> __TDO__RearRightShaft/7  "FrictionTrq[Nm]"
  FrictionTrq[Nm]___UNIQUE_1/1 -> __TDD__RearRightShaft.FrictionTrq[Nm]/1
  __TDD__RearRightShaft.AddInrt[kg*m**2]/1 -> __TDO__RearRightShaft/6  "AddInrt[kg*m**2]"
  AddInrt[kg*m**2]___UNIQUE_1/1 -> __TDD__RearRightShaft.AddInrt[kg*m**2]/1
  __TDD__RearRightShaft.DerivativeOfTrq_wrt_WheelSpd[Nm/(rad/s)]/1 -> __TDO__RearRightShaft/5  "DerivativeOfTrq_wrt_WheelSpd[Nm/(rad/s)]"
  DerivativeOfTrq_wrt_WheelSpd[Nm/(rad/s)]___UNIQUE_1/1 -> __TDD__RearRightShaft.DerivativeOfTrq_wrt_WheelSpd[Nm/(rad/s)]/1
  __TDD__RearRightShaft.DerivativeOfTrq_wrt_RotAng[Nm/rad]/1 -> __TDO__RearRightShaft/4  "DerivativeOfTrq_wrt_RotAng[Nm/rad]"
  DerivativeOfTrq_wrt_RotAng[Nm/rad]___UNIQUE_1/1 -> __TDD__RearRightShaft.DerivativeOfTrq_wrt_RotAng[Nm/rad]/1
  __TDD__RearRightShaft.RotAcc[rad/s**2]/1 -> __TDO__RearRightShaft/3  "RotAcc[rad/s**2]"
  RotAcc[rad/s**2]___UNIQUE_1/1 -> __TDD__RearRightShaft.RotAcc[rad/s**2]/1
  __TDD__RearRightShaft.RotSpdDifferentialOut[rad/s]/1 -> __TDO__RearRightShaft/2  "RotSpdDifferentialOut[rad/s]"
  RotSpdDifferentialOut[rad/s]___UNIQUE_1/1 -> __TDD__RearRightShaft.RotSpdDifferentialOut[rad/s]/1
  __TDD__RearRightShaft.Trq[Nm]/1 -> __TDO__RearRightShaft/1  "Trq[Nm]"
  Trq[Nm]___UNIQUE_1/1 -> __TDD__RearRightShaft.Trq[Nm]/1

== system SingleTrack/Vehicle/Drivetrain/DrivetrainPhysics/DrivetrainPhysicsOutputs/TransferCaseOutput/TransferCaseOutput ==
  TrqDistributionFac[0_1]___UNIQUE_1 : Inport  Description=|  PortDimensions=[1]
      | <name>TrqDistributionFac[0_1]</name>
      | <comment></comment>
  __TDD__TransferCase.TrqDistributionFac[0_1] : Demux  Outputs=[1]
  __TDO__TransferCase : BusCreator  Inputs=1
  TransferCase___UNIQUE_1 : Outport  Description=|  PortDimensions=[1]  VectorParamsAs1DForOutWhenUnconnected=off
      | <name>TrqDistributionFac[0_1]</name>
      | <comment></comment>
  wires:
  __TDO__TransferCase/1 -> TransferCase___UNIQUE_1/1  "TransferCase"
  __TDD__TransferCase.TrqDistributionFac[0_1]/1 -> __TDO__TransferCase/1  "TrqDistributionFac[0_1]"
  TrqDistributionFac[0_1]___UNIQUE_1/1 -> __TDD__TransferCase.TrqDistributionFac[0_1]/1

== system SingleTrack/Vehicle/Drivetrain/DrivetrainPhysics/DrivetrainPhysicsOutputs/TransmissionOutput/TransmissionOutput ==
  NumFwdGears[-]___UNIQUE_1 : Inport  Description=|  PortDimensions=[1]
      | <name>NumFwdGears[-]</name>
      | <comment></comment>
  Type[-]___UNIQUE_1 : Inport  Description=|  Port=2  PortDimensions=[1]
      | <name>Type[-]</name>
      | <comment></comment>
  Gear[-4;20]___UNIQUE_1 : Inport  Description=|  Port=3  PortDimensions=[1]
      | <name>Gear[-4;20]</name>
      | <comment></comment>
  InSpd[rad/s]___UNIQUE_1 : Inport  Description=|  Port=4  PortDimensions=[1]
      | <name>InSpd[rad/s]</name>
      | <comment></comment>
  OutSpd[rad/s]___UNIQUE_1 : Inport  Description=|  Port=5  PortDimensions=[1]
      | <name>OutSpd[rad/s]</name>
      | <comment></comment>
  GearChangeTimeConst[s]___UNIQUE_1 : Inport  Description=|  Port=6  PortDimensions=[1]
      | <name>GearChangeTimeConst[s]</name>
      | <comment></comment>
  __TDD__Transmission.GearChangeTimeConst[s] : Demux  Outputs=[1]
  __TDD__Transmission.Gear[-4;20] : Demux  Outputs=[1]
  __TDD__Transmission.InSpd[rad/s] : Demux  Outputs=[1]
  __TDD__Transmission.NumFwdGears[-] : Demux  Outputs=[1]
  __TDD__Transmission.OutSpd[rad/s] : Demux  Outputs=[1]
  __TDD__Transmission.Type[-] : Demux  Outputs=[1]
  __TDO__Transmission : BusCreator  Inputs=6
  Transmission___UNIQUE_1 : Outport  Description=|  PortDimensions=[6]  VectorParamsAs1DForOutWhenUnconnected=off
      | <name>NumFwdGears[-]</name>
      | <comment></comment>
  wires:
  __TDO__Transmission/1 -> Transmission___UNIQUE_1/1  "Transmission"
  __TDD__Transmission.GearChangeTimeConst[s]/1 -> __TDO__Transmission/6  "GearChangeTimeConst[s]"
  GearChangeTimeConst[s]___UNIQUE_1/1 -> __TDD__Transmission.GearChangeTimeConst[s]/1
  __TDD__Transmission.OutSpd[rad/s]/1 -> __TDO__Transmission/5  "OutSpd[rad/s]"
  OutSpd[rad/s]___UNIQUE_1/1 -> __TDD__Transmission.OutSpd[rad/s]/1
  __TDD__Transmission.InSpd[rad/s]/1 -> __TDO__Transmission/4  "InSpd[rad/s]"
  InSpd[rad/s]___UNIQUE_1/1 -> __TDD__Transmission.InSpd[rad/s]/1
  __TDD__Transmission.Gear[-4;20]/1 -> __TDO__Transmission/3  "Gear[-4;20]"
  Gear[-4;20]___UNIQUE_1/1 -> __TDD__Transmission.Gear[-4;20]/1
  __TDD__Transmission.Type[-]/1 -> __TDO__Transmission/2  "Type[-]"
  Type[-]___UNIQUE_1/1 -> __TDD__Transmission.Type[-]/1
  __TDD__Transmission.NumFwdGears[-]/1 -> __TDO__Transmission/1  "NumFwdGears[-]"
  NumFwdGears[-]___UNIQUE_1/1 -> __TDD__Transmission.NumFwdGears[-]/1

== system SingleTrack/VehicleControl/LateralControl/Disabled LateralControl/ControlSystems/Control Systems Parameters/CurvatureControl ==
  DynaModuleInfo : Subsystem  Tag=DynaModuleInfo
      mask init:
      | data = get_param(gcb, 'UserData');
      mask Display: disp(['Type = ', data.type, '\nName = ', char(data.name)]);

== system SingleTrack/VehicleControl/LateralControl/Disabled LateralControl/ControlSystems/Control Systems Parameters/PathControl ==
  DynaModuleInfo : Subsystem  Tag=DynaModuleInfo
      mask init:
      | data = get_param(gcb, 'UserData');
      mask Display: disp(['Type = ', data.type, '\nName = ', char(data.name)]);

== system SingleTrack/VehicleControl/LateralControl/Disabled LateralControl/ControlSystems/Lateral Controller/User-Defined Control ==
  UserDefinedControl : Subsystem
      settings: CopyFcn=DYNA4.Internal.ModelCallbacks.Modules.UpdateMaskParameters(gcb);  DeleteFcn=dm_close_block_mask  ModelCloseFcn=dm_close_block_mask  NameChangeFcn=DYNA4.Internal.ModelCallbacks.Modules.UpdateMaskParameters(gcb);  OpenFcn=dm_open_block_mask('vm_dflt_vehiclecontrol_user_defined_lateral_control');

== system SingleTrack/VehicleControl/LateralControl/Disabled LateralControl/ControlSystemsPreprocessor/Maneuver/DynaModuleInfo ==

== system SingleTrack/VehicleControl/LateralControl/Enabled LateralControl/ControlSystems/Lateral Controller/Initialization ==
  Action Port : ActionPort  InitializeStates=reset  PropagateVarSize=During execution  ActionPortLabel=default:
  Bus Creator : BusCreator  Inputs=3
  Constant : Constant  Value=0
  Constant1 : Constant  Value=0
  Constant2 : Constant  Value=0
  SteeringWheelDemands : Outport  VectorParamsAs1DForOutWhenUnconnected=off
  wires:
  Constant2/1 -> Bus Creator/3  "SteeringWheelInputSwitch[-]"
  Constant1/1 -> Bus Creator/2  "SteeringWheelTrq[Nm]"
  Bus Creator/1 -> SteeringWheelDemands/1
  Constant/1 -> Bus Creator/1  "SteeringWheelAng[rad]"

== system SingleTrack/VehicleControl/LateralControl/Enabled LateralControl/ControlSystems/Lateral Controller/Path and Curvature Control ==
  ControlInputs : Inport
  ControllerParameters : Inport  Port=2
  VehicleInfo : Inport  Port=3
  Action Port : ActionPort  InitializeStates=reset  PropagateVarSize=During execution  ActionPortLabel=case [ 3 4 ]:
  Bus Creator : BusCreator  Inputs=3
  Bus Selector1 : BusSelector  OutputSignals=Chassis_FrontAxle_Steering_SteeringWheelTrq[Nm]
  Constant1 : Constant  Value=0
  Gain : Gain
  PathControl : LateralControllerModules/PathControl  Tag=vedynaPathCtrlMask  local_comp_inst=1  system_comp_inst=1  sample_time=-1
  required by merge block : SignalConversion  OverrideOpt=off
  SteeringWheelDemands : Outport  VectorParamsAs1DForOutWhenUnconnected=off
  wires:
  Gain/1 -> Bus Creator/2  "SteeringWheelTrq[Nm]"
  Bus Selector1/1 -> Gain/1  "<Chassis_FrontAxle_Steering_SteeringWheelTrq[Nm]>"
  required by merge block/1 -> Bus Creator/1  "SteeringWheelAng[rad]"
  Constant1/1 -> Bus Creator/3  "SteeringWheelInputSwitch[-]"
  Bus Creator/1 -> SteeringWheelDemands/1
  PathControl/1 -> required by merge block/1
  ControllerParameters/1 -> PathControl/2
  ControlInputs/1 -> PathControl/1
  VehicleInfo/1 -> PathControl/3, Bus Selector1/1

== system SingleTrack/VehicleControl/LateralControl/Enabled LateralControl/ControlSystems/Lateral Controller/Steering Wheel Angle Input ==
  ControlInputs : Inport
  VehicleInfo : Inport  Port=2
  Action Port : ActionPort  InitializeStates=reset  PropagateVarSize=During execution  ActionPortLabel=case [ 1 ]:
  Bus Creator : BusCreator  Inputs=3
  Bus Selector : BusSelector  OutputSignals=SteeringWheelAng
  Bus Selector1 : BusSelector  OutputSignals=Chassis_FrontAxle_Steering_SteeringWheelTrq[Nm]
  Constant1 : Constant  Value=0
  Gain : Gain
  required by merge block : SignalConversion  OverrideOpt=off
  SteeringWheelDemands : Outport  VectorParamsAs1DForOutWhenUnconnected=off
  wires:
  Gain/1 -> Bus Creator/2  "SteeringWheelTrq[Nm]"
  VehicleInfo/1 -> Bus Selector1/1
  Constant1/1 -> Bus Creator/3  "SteeringWheelInputSwitch[-]"
  Bus Selector1/1 -> Gain/1  "<Chassis_FrontAxle_Steering_SteeringWheelTrq[Nm]>"
  Bus Creator/1 -> SteeringWheelDemands/1
  required by merge block/1 -> Bus Creator/1  "SteeringWheelAng[rad]"
  Bus Selector/1 -> required by merge block/1  "<SteeringWheelAng>"
  ControlInputs/1 -> Bus Selector/1

== system SingleTrack/VehicleControl/LateralControl/Enabled LateralControl/ControlSystems/Lateral Controller/Steering Wheel Torque Input ==
  ControlInputs : Inport
  VehicleInfo : Inport  Port=2
  Action Port : ActionPort  InitializeStates=reset  PropagateVarSize=During execution  ActionPortLabel=case [ 2 ]:
  Bus Creator : BusCreator  Inputs=3
  Bus Selector : BusSelector  OutputSignals=SteeringWheelTrq
  Bus Selector1 : BusSelector  OutputSignals=Chassis_FrontAxle_Steering_SteeringWheelAng[rad]
  Constant1 : Constant
  Gain : Gain
  required by merge block : SignalConversion  OverrideOpt=off
  SteeringWheelDemands : Outport  VectorParamsAs1DForOutWhenUnconnected=off
  wires:
  Gain/1 -> Bus Creator/1  "SteeringWheelAng[rad]"
  required by merge block/1 -> Bus Creator/2  "SteeringWheelTrq[Nm]"
  VehicleInfo/1 -> Bus Selector1/1
  Bus Selector/1 -> required by merge block/1  "<SteeringWheelTrq>"
  ControlInputs/1 -> Bus Selector/1
  Bus Selector1/1 -> Gain/1  "<Chassis_FrontAxle_Steering_SteeringWheelAng[rad]>"
  Bus Creator/1 -> SteeringWheelDemands/1
  Constant1/1 -> Bus Creator/3  "SteeringWheelInputSwitch[-]"

== system SingleTrack/VehicleControl/LateralControl/Enabled LateralControl/ControlSystems/Lateral Controller/User-Defined Control ==
  ControlInputs : Inport
  VehicleInfo : Inport  Port=2
  SourceIdentifiers : Inport  Port=3
  SubtaskIdentifiers : Inport  Port=4
  Action Port : ActionPort  InitializeStates=reset  PropagateVarSize=During execution  ActionPortLabel=case [ 5 ]:
  Bus Creator : BusCreator  Inputs=3
  Bus Selector1 : BusSelector  OutputSignals=UserDefinedRefValue
  Bus Selector2 : BusSelector  OutputSignals=Chassis_FrontAxle_Steering_SteeringWheelTrq[Nm]
  Constant1 : Constant  Value=0
  Gain : Gain
  UserDefinedControl : LateralControllerModules/UserDefinedLateralControl  DATA_NODE=MDL.VehicleControl.LateralControl.ControlSystems.UserDefinedControl  SteeringWheelAngle=MDL.VehicleControl.LateralControl.ControlSystems.UserDefinedControl.SteeringWheelAng
  SteeringWheelDemands : Outport  VectorParamsAs1DForOutWhenUnconnected=off
  UserDefinedRefValue[-] : Outport  Port=2  PortDimensions=1  OutputWhenDisabled=reset  InitialOutput=0  VectorParamsAs1DForOutWhenUnconnected=off
  wires:
  Gain/1 -> Bus Creator/2  "SteeringWheelTrq[Nm]"
  Bus Selector2/1 -> Gain/1  "<Chassis_FrontAxle_Steering_SteeringWheelTrq[Nm]>"
  Constant1/1 -> Bus Creator/3  "SteeringWheelInputSwitch[-]"
  Bus Creator/1 -> SteeringWheelDemands/1
  UserDefinedControl/1 -> Bus Creator/1  "SteeringWheelAng[rad]"
  Bus Selector1/1 -> UserDefinedRefValue[-]/1  "<UserDefinedRefValue>"
  SubtaskIdentifiers/1 -> UserDefinedControl/1
  VehicleInfo/1 -> UserDefinedControl/4, Bus Selector2/1
  SourceIdentifiers/1 -> UserDefinedControl/2
  ControlInputs/1 -> Bus Selector1/1, UserDefinedControl/3

== system SingleTrack/VehicleControl/LateralControl/Enabled LateralControl/ControlSystemsPreprocessor/External Presetting of Controller /Presetting Source Identifiers ==
  note: SOURCE_NOMINALPATH = 1;
      | 	SOURCE_LANE = 2;
      | 	SOURCE_CONSTANT = 3;
      | 	SOURCE_TABLE_DISCRETE = 4;
      | 	SOURCE_TABLE_LINEAR = 5;
      | 	SOURCE_TABLE_CUBIC = 6;
      | 	SOURCE_TABLE_HAVERSINE = 7;
      | 	SOURCE_AUTOMATIC = 8;
      | 	SOURCE_SINE_TIME = 9;
      | 	SOURCE_SINE_PATH = 10;
      | 	SOURCE_HOLD = 11;
      | 	SOURCE_EXTERNAL = 12;
      | 	SOURCE_EXTERNAL_NOMINALPATH = 13;
      | 	SOURCE_EXTERNAL_LANE = 14;
  "ExternalControlVariablesEnforced " : Inport
  SourceIdentifiers : Inport  Port=2
  Bus Selector : BusSelector  OutputSignals=CTRL_LateralControl_RefPathEnforced,CTRL_LateralControl_RefLaneEnforced,CTRL_LateralControl_RefLatPosEnforced,CTRL_LateralControl_RefCurvEnforced,CTRL_LateralControl_UserDefinedRefValueEnforced
  Bus Selector6 : BusSelector  OutputSignals=RefPath,RefLane,RefLatPos,RefPathCurv,UserDefinedRefValue
  PathCtrl_Path : BusAssignment  AssignedSignals=RefPath,RefLane,RefLatPos,RefPathCurv,UserDefinedRefValue
  RefLaneExternal : Constant  Value=vm_const('SOURCE_EXTERNAL_LANE')
  RefLatPosExternal : Constant  Value=vm_const('SOURCE_EXTERNAL')
  RefPathCurvExternal : Constant  Value=vm_const('SOURCE_EXTERNAL')
  RefPathExternal : Constant  Value=vm_const('SOURCE_EXTERNAL_NOMINALPATH')
  Switch{1..2,5..7} (5 alike) : Switch  Criteria=u2 > Threshold
  UserDefinedRefValueExternal : Constant  Value=vm_const('SOURCE_EXTERNAL')
  ModifiedSourceIdentifiers : Outport  VectorParamsAs1DForOutWhenUnconnected=off
  wires:
  Bus Selector6/5 -> Switch2/3  "<UserDefinedRefValue>"
  Bus Selector6/4 -> Switch1/3  "<RefPathCurv>"
  Bus Selector6/3 -> Switch7/3  "<RefLatPos>"
  Bus Selector6/2 -> Switch6/3  "<RefLane>"
  Bus Selector6/1 -> Switch5/3  "<RefPath>"
  Switch2/1 -> PathCtrl_Path/6
  Switch1/1 -> PathCtrl_Path/5
  Switch7/1 -> PathCtrl_Path/4
  Switch6/1 -> PathCtrl_Path/3
  Switch5/1 -> PathCtrl_Path/2
  PathCtrl_Path/1 -> ModifiedSourceIdentifiers/1
  Bus Selector/5 -> Switch2/2  "<CTRL_LateralControl_UserDefinedRefValueEnforced>"
  UserDefinedRefValueExternal/1 -> Switch2/1
  RefPathCurvExternal/1 -> Switch1/1
  Bus Selector/4 -> Switch1/2  "<CTRL_LateralControl_RefCurvEnforced>"
  RefLatPosExternal/1 -> Switch7/1
  Bus Selector/3 -> Switch7/2  "<CTRL_LateralControl_RefLatPosEnforced>"
  Bus Selector/2 -> Switch6/2  "<CTRL_LateralControl_RefLaneEnforced>"
  RefLaneExternal/1 -> Switch6/1
  RefPathExternal/1 -> Switch5/1
  Bus Selector/1 -> Switch5/2  "<CTRL_LateralControl_RefPathEnforced>"
  "ExternalControlVariablesEnforced "/1 -> Bus Selector/1
  SourceIdentifiers/1 -> PathCtrl_Path/1, Bus Selector6/1

== system SingleTrack/VehicleControl/LateralControl/Enabled LateralControl/ControlSystemsPreprocessor/External Presetting of Controller /Presetting Task Identifiers ==
  TaskIdentifiers : Inport
  "ExternalControlVariablesEnforced " : Inport  Port=2
  Bus Creator : BusCreator  Inputs=2
  Bus Selector : BusSelector  OutputSignals=CTRL_LateralControl_RefPathEnforced,CTRL_LateralControl_RefLaneEnforced,CTRL_LateralControl_RefLatPosEnforced,CTRL_LateralControl_RefCurvEnforced,CTRL_LateralControl_UserDefinedRefValueEnforced  OutputAsBus=on
  Bus Selector1 : BusSelector  OutputSignals=Task[-],Subtask[-]
  Bus to Vector : BusToVector
  ChooseMax : MinMax  Function=max
  Demux : Demux  Outputs=2
  Gain : Gain  Gain=[5 4 3 2 1]
  Multiport Switch : MultiPortSwitch  DataPortOrder=Zero-based contiguous  Inputs=6  zeroidx=on
  Mux : Mux  Inputs=2
  Speed Control : Constant  Value=[vm_const('TASK_LAT_PATH_CONTROL') vm_const('SUBTASK_LAT_PATH_CONTROL_PATH')]
  Speed Control1 : Constant  Value=[vm_const('TASK_LAT_CURVATURE_CONTROL') 0]
  Speed Control2 : Constant  Value=[vm_const('TASK_LAT_USER_DEFINED') 0]
  Speed Control3 : Constant  Value=[vm_const('TASK_LAT_PATH_CONTROL') vm_const('SUBTASK_LAT_PATH_CONTROL_LANE')]
  Speed Control4 : Constant  Value=[vm_const('TASK_LAT_PATH_CONTROL') vm_const('SUBTASK_LAT_PATH_CONTROL_LATERAL_POS')]
  ModifiedTaskIdentifiers : Outport  VectorParamsAs1DForOutWhenUnconnected=off
  wires:
  Multiport Switch/1 -> Demux/1
  Speed Control2/1 -> Multiport Switch/3
  Speed Control1/1 -> Multiport Switch/4
  Speed Control4/1 -> Multiport Switch/5
  Speed Control3/1 -> Multiport Switch/6
  Speed Control/1 -> Multiport Switch/7
  Mux/1 -> Multiport Switch/2
  Gain/1 -> ChooseMax/1
  Bus to Vector/1 -> Gain/1
  Bus Selector/1 -> Bus to Vector/1
  Bus Selector1/1 -> Mux/1  "<Task[-]>"
  Bus Selector1/2 -> Mux/2  "<Subtask[-]>"
  "ExternalControlVariablesEnforced "/1 -> Bus Selector/1
  TaskIdentifiers/1 -> Bus Selector1/1
  Bus Creator/1 -> ModifiedTaskIdentifiers/1
  Demux/1 -> Bus Creator/1  "Task"
  Demux/2 -> Bus Creator/2  "Subtask"
  ChooseMax/1 -> Multiport Switch/1  "switch value"

== system SingleTrack/VehicleControl/LateralControl/Enabled LateralControl/ControlSystemsPreprocessor/Generation of Guidance Data/Initialization, SteeringWheel, UserDefined ==
  Action Port : ActionPort  InitializeStates=reset  ActionPortLabel=default:
  Constant : Constant  Value=zeros(1,7)
  TargetAndTargetAim : Outport  VectorParamsAs1DForOutWhenUnconnected=off
  wires:
  Constant/1 -> TargetAndTargetAim/1

== system SingleTrack/VehicleControl/LateralControl/Enabled LateralControl/ControlSystemsPreprocessor/Generation of Hold Data/Enabled Subsystem ==
  LatCTRL : Inport
  VehicleInfo : Inport  Port=2
  Enable : EnablePort  StatesWhenEnabling=reset  PropagateVarSize=During execution
  Bus Assignment : BusAssignment  AssignedSignals=SteeringWheelAng,SteeringWheelTrq,LeftIndicator,RightIndicator,RefLatPos,RefLane,RefPathCurv
  Bus Selector18 : BusSelector  OutputSignals=VehicleRoadInfo_RoadQ[m],VehicleRoadInfo_LaneID[-],VehicleRoadInfo_LaneCurvature[1/m]
  Bus Selector8 : BusSelector  OutputSignals=SteeringWheelAng[rad],SteeringWheelTrq[Nm],LeftIndicator[0;1],RightIndicator[0;1]
  TD_BO_LateralControlInputs all zeros : Constant  Value=0  OutDataTypeStr=Bus: TD_BO_LateralControlInputs
  HoldData : Outport  VectorParamsAs1DForOutWhenUnconnected=off
  wires:
  Bus Selector18/2 -> Bus Assignment/7  "<VehicleRoadInfo_LaneID[-]>"
  Bus Selector18/3 -> Bus Assignment/8  "<VehicleRoadInfo_LaneCurvature[1/m]>"
  Bus Selector18/1 -> Bus Assignment/6  "<VehicleRoadInfo_RoadQ[m]>"
  Bus Selector8/4 -> Bus Assignment/5  "<RightIndicator[0;1]>"
  Bus Selector8/3 -> Bus Assignment/4  "<LeftIndicator[0;1]>"
  Bus Selector8/2 -> Bus Assignment/3  "<SteeringWheelTrq[Nm]>"
  Bus Assignment/1 -> HoldData/1
  TD_BO_LateralControlInputs all zeros/1 -> Bus Assignment/1
  VehicleInfo/1 -> Bus Selector18/1
  LatCTRL/1 -> Bus Selector8/1
  Bus Selector8/1 -> Bus Assignment/2  "<SteeringWheelAng[rad]>"

== system SingleTrack/VehicleControl/LongitudinalControl/ControlSystems/Longitudinal Controller/Acceleration Control/ComputeBrakePedalPos ==
  VehicleInfo : Inport
  RefTireTrq[Nm] : Inport  Port=2
  Bus Selector : BusSelector  OutputSignals=VehicleDriverInfo_AccPedalPos[0_1]
  Calculate Brake Pedal : Subsystem
  Constant1 : Constant  Value=0
  Factor_TyreTorque_2_BrakePedalPosition : Subsystem
  no Brake AND Gas : Subsystem
  BrakePedalPos[0_1] : Outport  VectorParamsAs1DForOutWhenUnconnected=off
  wires:
  Bus Selector/1 -> no Brake AND Gas/1(AccPedal)  "<VehicleDriverInfo_AccPedalPos[0_1]>"
  VehicleInfo/1 -> Factor_TyreTorque_2_BrakePedalPosition/1(VehicleInfo), Bus Selector/1
  RefTireTrq[Nm]/1 -> Calculate Brake Pedal/2(Int Torque on Wheel)
  no Brake AND Gas/1(ModifiedBrakePedalPos [0-1]) -> BrakePedalPos[0_1]/1
  Constant1/1 -> no Brake AND Gas/3(PedalChangeTime)  "<MinPedalChangeTime[s]>"
  Calculate Brake Pedal/1(Brake Pedal Position) -> no Brake AND Gas/2(BrakePedal)
  Factor_TyreTorque_2_BrakePedalPosition/1(Factor_TyreTorque_2_BrakePedalPosition) -> Calculate Brake Pedal/1(Factor_TyreTorque_2_BrakePedalPosition)

== system SingleTrack/VehicleControl/LongitudinalControl/ControlSystems/Longitudinal Controller/Acceleration Control/ComputeIntEngTrq ==
  FeedforwardTrq[Nm] : Inport
  VehicleInfo : Inport  Port=2
  ControlTrq[Nm] : Inport  Port=3
  Avoid_Zero : Saturate  UpperLimit=inf  LowerLimit=0.1
  Bus Selector : BusSelector  OutputSignals=VehicleDriverInfo_TorqueRatio[-]
  Divide : Product  Inputs=*/
  IntTrqWheel : Sum
  Memory1 : Memory  InheritSampleTime=on
  RefTireTrq[Nm] : Outport  VectorParamsAs1DForOutWhenUnconnected=off
  RefEngTrq[Nm] : Outport  Port=2  VectorParamsAs1DForOutWhenUnconnected=off
  wires:
  Memory1/1 -> Divide/1, RefTireTrq[Nm]/1
  Avoid_Zero/1 -> Divide/2
  IntTrqWheel/1 -> Memory1/1
  Divide/1 -> RefEngTrq[Nm]/1
  Bus Selector/1 -> Avoid_Zero/1  "<VehicleDriverInfo_TorqueRatio[-]>"
  ControlTrq[Nm]/1 -> IntTrqWheel/2
  FeedforwardTrq[Nm]/1 -> IntTrqWheel/1
  VehicleInfo/1 -> Bus Selector/1

== system SingleTrack/VehicleControl/LongitudinalControl/ControlSystems/Longitudinal Controller/Acceleration Control/Write To ControlOutputs ==
  BrakePedalPos[0_1] : Inport
  IntendedEngTrq[Nm] : Inport  Port=2
  EngSpd[rad/s] : Inport  Port=3
  RefAcc[rad/s] : Inport  Port=4
  Bus Assignment : BusAssignment  AssignedSignals=BrakePedalPos,IntendedEngTrq,EngSpd,RefAcc
  Create SpeedControlOutput Bus : Constant  Value=0  OutDataTypeStr=Bus: TD_BO_LongitudinalSpeedControlOutputs
  ControlOutputs : Outport  VectorParamsAs1DForOutWhenUnconnected=off
  wires:
  Bus Assignment/1 -> ControlOutputs/1
  Create SpeedControlOutput Bus/1 -> Bus Assignment/1
  BrakePedalPos[0_1]/1 -> Bus Assignment/2
  RefAcc[rad/s]/1 -> Bus Assignment/5  "RefAcc[m/s**2]"
  EngSpd[rad/s]/1 -> Bus Assignment/4  "EngSpd[rad/s]"
  IntendedEngTrq[Nm]/1 -> Bus Assignment/3  "IntendedEngTrq[Nm]"

== system SingleTrack/VehicleControl/LongitudinalControl/ControlSystems/Longitudinal Controller/Compute Acc Pedal Position/Invert Acc Pedal ==
  VehicleInfo : Inport
  ControlOutputs : Inport  Port=2
  Action Port : ActionPort  InitializeStates=reset  PropagateVarSize=During execution  ActionPortLabel=case [ 0 2 3 4 ]:
  InvAccPedal : LongitudinalControllerModules/InvAccPedal  Tag=vedynaInvAccPedalMask  SystemSampleTime=-1  Latency=0  AutoFrameSizeCalculation=off
  ModifiedControlOutputs : Outport  VectorParamsAs1DForOutWhenUnconnected=off
  wires:
  InvAccPedal/1 -> ModifiedControlOutputs/1
  VehicleInfo/1 -> InvAccPedal/1
  ControlOutputs/1 -> InvAccPedal/2

== system SingleTrack/VehicleControl/LongitudinalControl/ControlSystems/Longitudinal Controller/Compute Acc Pedal Position/Pass Through ControlOutputs ==
  ControlOutputs : Inport
  Action Port : ActionPort  InitializeStates=reset  PropagateVarSize=During execution  ActionPortLabel=case [ 1 ]:
  ModifiedControlOutputs : Outport  VectorParamsAs1DForOutWhenUnconnected=off
  wires:
  ControlOutputs/1 -> ModifiedControlOutputs/1
